simulink model "EPS_orbit_v1_R2019a"  (R2019a)
settings: Solver=FixedStepAuto  StartTime=0.0  StopTime=tsimulation  FixedStep=delta_t  RelTol=1e-3
values from neighbouring files (symbols this model uses):
  a = 6678    [demoEPS_R2019a.m]    (also in demoEPS_v1.m; demoEPS_v1a.m; demoEPS_v1test.m; demoEPS_v2.m)
  day = 21    [demoEPS_R2019a.m]    (also in demoEPS_v1.m = 1; demoEPS_v1a.m; demoEPS_v1test.m; demoEPS_v2.m)
  e = 0.001    [demoEPS_R2019a.m]    (also in demoEPS_v1.m = 0; demoEPS_v1a.m; demoEPS_v1test.m; demoEPS_v2.m)
  hours = 0    [demoEPS_R2019a.m]    (also in demoEPS_v1.m; demoEPS_v1a.m; demoEPS_v1test.m; demoEPS_v2.m)
  i = 51.6    [demoEPS_R2019a.m]    (also in demoEPS_v1.m; demoEPS_v1a.m; demoEPS_v1test.m; demoEPS_v2.m)
  m = 10    [demoEPS_R2019a.m]    (also in demoEPS_v1.m; demoEPS_v1a.m; demoEPS_v1test.m; demoEPS_v2.m)
  minutes = 0    [demoEPS_R2019a.m]    (also in demoEPS_v1.m; demoEPS_v1a.m; demoEPS_v1test.m; demoEPS_v2.m)
  month = 3    [demoEPS_R2019a.m]    (also in demoEPS_v1.m = 1; demoEPS_v1a.m = 6; demoEPS_v1test.m = 12; demoEPS_v2.m)
  nu = 0    [demoEPS_R2019a.m]    (also in demoEPS_v1.m; demoEPS_v1a.m; demoEPS_v1test.m; demoEPS_v2.m)
  O = 300    [demoEPS_R2019a.m]    (also in demoEPS_v1.m = 185; demoEPS_v1a.m = 69; demoEPS_v1test.m = 180; demoEPS_v2.m = 243)
  o = 90    [demoEPS_R2019a.m]    (also in demoEPS_v1.m; demoEPS_v1a.m = 150; demoEPS_v1test.m = 150; demoEPS_v2.m)
  Psa = 48    [demoEPS.m]    (also in demoEPS_R2019a.m; demoEPS_v1.m; demoEPS_v1a.m; demoEPS_v1test.m)
  seconds = 0    [demoEPS_R2019a.m]    (also in demoEPS_v1.m; demoEPS_v1a.m; demoEPS_v1test.m; demoEPS_v2.m)
  year = 2020    [demoEPS_R2019a.m]    (also in demoEPS_v1.m; demoEPS_v1a.m = 2019; demoEPS_v1test.m = 2019; demoEPS_v2.m)
undefined symbols (not defined in the file or in its folder): km, s
libraries: aerolibconvert2 x6, vrlib x5, dspmathops x2, aerolibutil x2, sharedtransform x1, aerolibgravity2 x1, aerolibcelestial x1
settings Model: Creator=Ricardo  LastModifiedBy=colpari

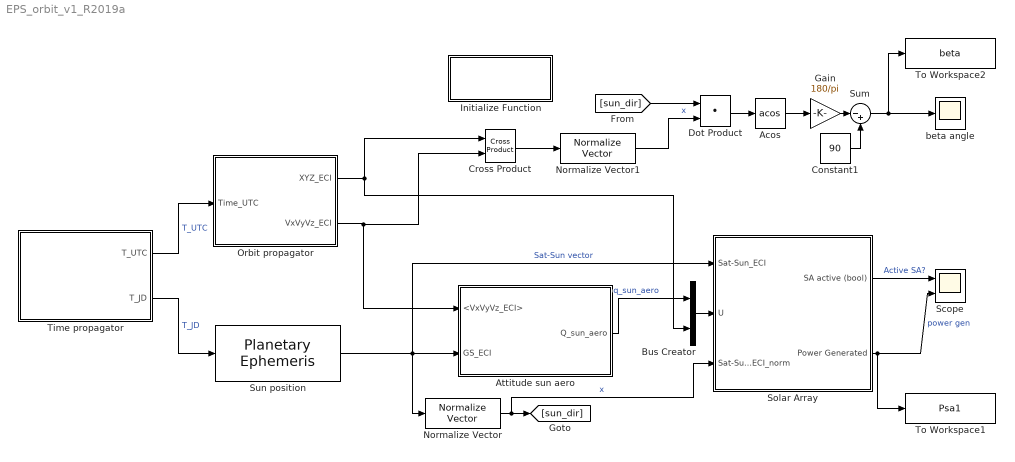
== system EPS_orbit_v1_R2019a ==
  Acos : Trigonometry  Operator=acos
  Attitude sun aero : Subsystem
  Bus Creator : BusCreator  Inputs=2
  Constant1 : Constant  Value=90
  Cross Product : vrlib/Utilities/Cross Product
  Dot Product : DotProduct  InputSameDT=on  OutDataTypeStr=Inherit: Inherit via internal rule
  Gain : Gain  Gain=180/pi
  Initialize Function : Subsystem  TreatAsAtomicUnit=on
  Normalize Vector : vrlib/Utilities/Normalize Vector  maxzero=0
  Normalize Vector1 : vrlib/Utilities/Normalize Vector  maxzero=0
  Orbit propagator : Subsystem
  Scope : Scope  NumInputPorts=2
  Solar Array : Subsystem
  Sum : Sum  Inputs=|-+
  Sun position : aerolibcelestial/Planetary Ephemeris  kmflag=km,km/s  epochflag=Julian date  de=DE405  nCenter=Earth  nTarget=Sun  errorflag=Error  velflag=off
      settings: SourceProductBaseCode=AE
  Time propagator : Subsystem
  To Workspace1 : ToWorkspace  VariableName=Psa1  SaveFormat=Timeseries  SampleTime=-1
  To Workspace2 : ToWorkspace  VariableName=beta  SaveFormat=Timeseries  SampleTime=-1
  beta angle : Scope
  wires:
  Orbit propagator/2(VxVyVz_ECI) -> Cross Product/2, Attitude sun aero/1(<VxVyVz_ECI>)
  Orbit propagator/1(XYZ_ECI) -> Cross Product/1, Bus Creator/2
  Normalize Vector/1 -> [sun_dir], Solar Array/3(Sat-Sun_ECI_norm)  "x"
  Bus Creator/1 -> Solar Array/2(U)
  Sun position/1 -> Normalize Vector/1, Solar Array/1(Sat-Sun_ECI), Attitude sun aero/2(GS_ECI)  "Sat-Sun vector"
  Solar Array/1(SA active (bool)) -> Scope/1  "Active SA?"
  Time propagator/1(T_UTC) -> Orbit propagator/1("Time_UTC ")  "T_UTC"
  Attitude sun aero/1(Q_sun_aero) -> Bus Creator/1  "q_sun_aero"
  Normalize Vector1/1 -> Dot Product/2  "x"
  Gain/1 -> Sum/1
  Solar Array/2(Power Generated) -> To Workspace1/1, Scope/2  "power gen"
  [sun_dir] -> Dot Product/1
  Acos/1 -> Gain/1
  Dot Product/1 -> Acos/1
  Time propagator/2(T_JD) -> Sun position/1  "T_JD"
  Cross Product/1 -> Normalize Vector1/1
  Sum/1 -> beta angle/1, To Workspace2/1
  Constant1/1 -> Sum/2

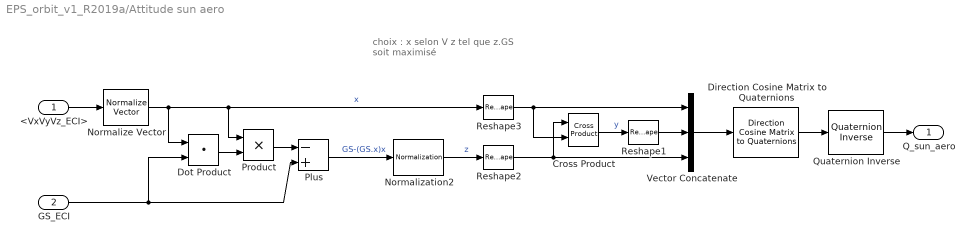
== system EPS_orbit_v1_R2019a/Attitude sun aero ==
  note: choix :
      | x selon V
      | z tel que z.GS soit maximisé
  <VxVyVz_ECI> : Inport
  GS_ECI : Inport  Port=2
  Cross Product : vrlib/Utilities/Cross Product
  Direction Cosine Matrix to Quaternions : sharedtransform/Direction Cosine Matrix  to Quaternions  aMode=0  action=None  tolerance=eps(2)
      settings: SourceProductBaseCode=AE,PW,MT,UV,VE,VP
  Dot Product : DotProduct  InputSameDT=on  OutDataTypeStr=Inherit: Inherit via internal rule
  Normalization2 : dspmathops/Normalization  NormType=2-norm  Bias=1e-10  NormOver=Each column  Dimension=1  roundingMode=Floor  overflowMode=off  accumDataTypeStr=Inherit: Same as product output  accumLastDataTypeStr=Inherit: Same as product output  outputDataTypeStr=Inherit: Same as product output  outputMin=[]  outputMax=[]  outputLastDataTypeStr=Inherit: Same as product output
  Normalize Vector : vrlib/Utilities/Normalize Vector  maxzero=0
  Plus : Sum  Inputs=-+
  Product : Product
  Quaternion Inverse : aerolibutil/Quaternion Inverse
  Reshape1 : Reshape  OutputDimensionality=Column vector (2-D)
  Reshape2 : Reshape  OutputDimensionality=Column vector (2-D)
  Reshape3 : Reshape  OutputDimensionality=Column vector (2-D)
  Vector Concatenate : Concatenate  NumInputs=3  Mode=Multidimensional array  ConcatenateDimension=2
  Q_sun_aero : Outport  VectorParamsAs1DForOutWhenUnconnected=off
  wires:
  Quaternion Inverse/1 -> Q_sun_aero/1
  Reshape2/1 -> Vector Concatenate/3, Cross Product/1
  Reshape3/1 -> Vector Concatenate/1, Cross Product/2
  Product/1 -> Plus/1
  Dot Product/1 -> Product/2
  Cross Product/1 -> Reshape1/1  "y"
  Normalization2/1 -> Reshape2/1  "z"
  Plus/1 -> Normalization2/1  "GS-(GS.x)x"
  GS_ECI/1 -> Dot Product/2, Plus/2
  Vector Concatenate/1 -> Direction Cosine Matrix to Quaternions/1
  Direction Cosine Matrix to Quaternions/1 -> Quaternion Inverse/1
  Normalize Vector/1 -> Dot Product/1, Product/1, Reshape3/1  "x"
  <VxVyVz_ECI>/1 -> Normalize Vector/1
  Reshape1/1 -> Vector Concatenate/2

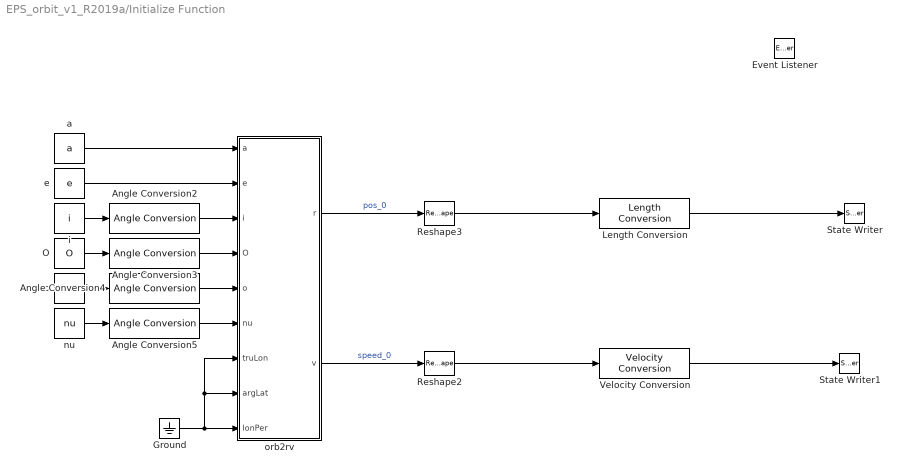
== system EPS_orbit_v1_R2019a/Initialize Function ==
  Angle Conversion{2..5} (4 alike) : aerolibconvert2/Angle Conversion  IU=deg  OU=rad
  Event Listener : EventListener  DisableCoverage=on  EventName=reset
  Ground : Ground
  Length Conversion : aerolibconvert2/Length Conversion  IU=km  OU=m
  O : Constant  Value=O
  Reshape2 : Reshape  OutputDimensionality=Column vector (2-D)
  Reshape3 : Reshape  OutputDimensionality=Column vector (2-D)
  State Writer : StateWriter  StateOwnerBlock=../../Orbit propagator/Integrator_pos
  State Writer1 : StateWriter  StateOwnerBlock=../../Orbit propagator/Integrator_speed
  Velocity Conversion : aerolibconvert2/Velocity Conversion  IU=km/s  OU=m/s
  a : Constant  Value=a
  e : Constant  Value=e
  i : Constant  Value=i
  nu : Constant  Value=nu
  o : Constant  Value=o
  orb2rv : MATLAB Function  TreatAsAtomicUnit=on
  wires:
  Angle Conversion2/1 -> orb2rv/3(i)
  Length Conversion/1 -> State Writer/1
  Angle Conversion4/1 -> orb2rv/5(o)
  nu/1 -> Angle Conversion5/1
  Angle Conversion3/1 -> orb2rv/4(O)
  e/1 -> orb2rv/2(e)
  Reshape3/1 -> Length Conversion/1
  O/1 -> Angle Conversion3/1
  a/1 -> orb2rv/1(a)
  i/1 -> Angle Conversion2/1
  orb2rv/1(r) -> Reshape3/1  "pos_0"
  o/1 -> Angle Conversion4/1
  Angle Conversion5/1 -> orb2rv/6(nu)
  Velocity Conversion/1 -> State Writer1/1
  Reshape2/1 -> Velocity Conversion/1
  orb2rv/2(v) -> Reshape2/1  "speed_0"
  Ground/1 -> orb2rv/8(argLat), orb2rv/7(truLon), orb2rv/9(lonPer)

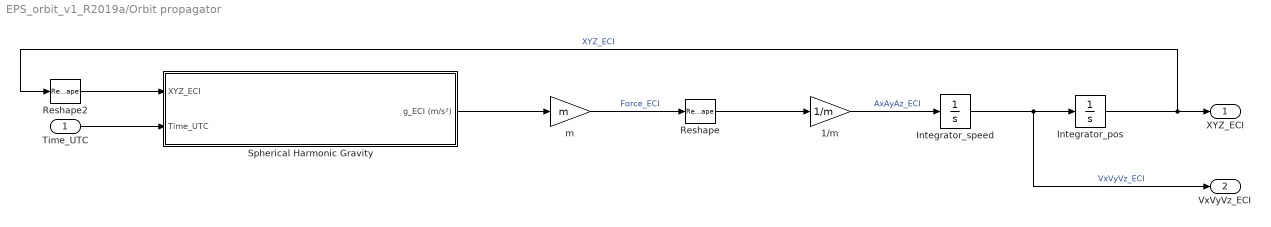
== system EPS_orbit_v1_R2019a/Orbit propagator ==
  "Time_UTC " : Inport
  1/m : Gain  Gain=1/m
  Integrator_pos : Integrator
  Integrator_speed : Integrator
  Reshape : Reshape  OutputDimensionality=Column vector (2-D)
  Reshape2 : Reshape  OutputDimensionality=Column vector (2-D)
  Spherical Harmonic Gravity : Subsystem  TreatAsAtomicUnit=on  SystemSampleTime=1
  m : Gain  Gain=m
  XYZ_ECI : Outport  VectorParamsAs1DForOutWhenUnconnected=off
  VxVyVz_ECI : Outport  Port=2
  wires:
  Integrator_pos/1 -> Reshape2/1, XYZ_ECI/1  "XYZ_ECI"
  Integrator_speed/1 -> VxVyVz_ECI/1, Integrator_pos/1  "VxVyVz_ECI"
  1/m/1 -> Integrator_speed/1  "AxAyAz_ECI"
  Reshape/1 -> 1/m/1
  m/1 -> Reshape/1  "Force_ECI"
  Spherical Harmonic Gravity/1(g_ECI (m/s²)) -> m/1
  "Time_UTC "/1 -> Spherical Harmonic Gravity/2(Time_UTC)
  Reshape2/1 -> Spherical Harmonic Gravity/1(XYZ_ECI)

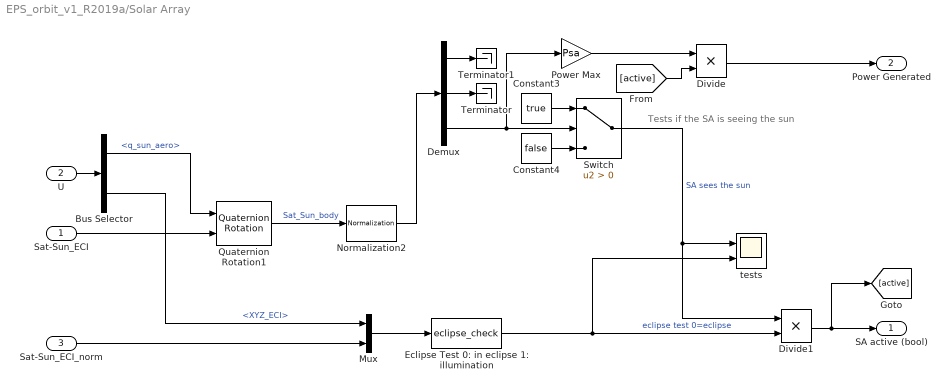
== system EPS_orbit_v1_R2019a/Solar Array ==
  note: Tests if the SA is seeing the sun
  Sat-Sun_ECI : Inport
  U : Inport  Port=2
  Sat-Sun_ECI_norm : Inport  Port=3
  Bus Selector : BusSelector  OutputSignals=q_sun_aero,XYZ_ECI
  Constant3 : Constant  Value=true
  Constant4 : Constant  Value=false
  Demux : Demux  Outputs=3
  Divide : Product  Inputs=**
  Divide1 : Product  Inputs=**
  Eclipse Test 0: in eclipse 1: illumination : MATLABFcn  MATLABFcn=eclipse_check
  Mux : Mux  Inputs=2
  Normalization2 : dspmathops/Normalization  NormType=2-norm  Bias=1e-10  NormOver=Each column  Dimension=1  roundingMode=Floor  overflowMode=off  accumDataTypeStr=Inherit: Same as product output  accumLastDataTypeStr=Inherit: Same as product output  outputDataTypeStr=Inherit: Same as product output  outputMin=[]  outputMax=[]  outputLastDataTypeStr=Inherit: Same as product output
  Power Max : Gain  Gain=Psa
  Quaternion Rotation1 : aerolibutil/Quaternion Rotation
  Switch : Switch  Criteria=u2 > Threshold
  Terminator : Terminator
  Terminator1 : Terminator
  tests : Scope  NumInputPorts=2
  SA active (bool) : Outport  VectorParamsAs1DForOutWhenUnconnected=off
  Power Generated : Outport  Port=2
  wires:
  Switch/1 -> Divide1/1, tests/1  "SA sees the sun"
  U/1 -> Bus Selector/1
  Sat-Sun_ECI/1 -> Quaternion Rotation1/2
  Bus Selector/1 -> Quaternion Rotation1/1  "<q_sun_aero>"
  Quaternion Rotation1/1 -> Normalization2/1  "Sat_Sun_body"
  Demux/3 -> Power Max/1, Switch/2
  Constant3/1 -> Switch/1
  Demux/2 -> Terminator/1
  Demux/1 -> Terminator1/1
  Bus Selector/2 -> Mux/1  "<XYZ_ECI>"
  Divide1/1 -> [active], SA active (bool)/1
  Constant4/1 -> Switch/3
  Normalization2/1 -> Demux/1
  Divide/1 -> Power Generated/1
  Power Max/1 -> Divide/1
  [active] -> Divide/2
  Sat-Sun_ECI_norm/1 -> Mux/2
  Mux/1 -> Eclipse Test 0: in eclipse 1: illumination/1
  Eclipse Test 0: in eclipse 1: illumination/1 -> tests/2, Divide1/2  "eclipse test 0=eclipse"

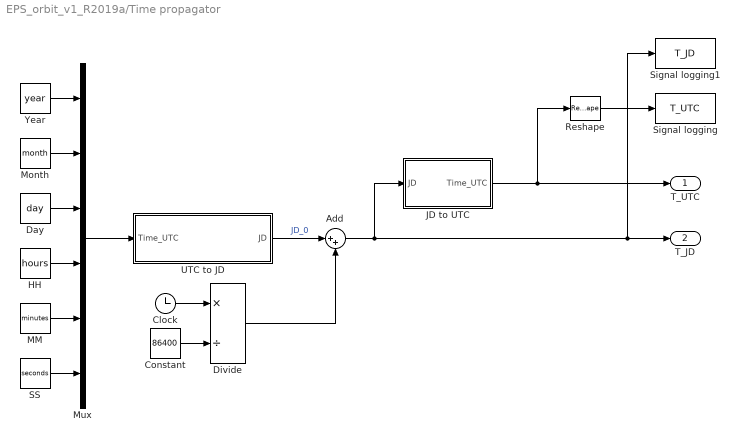
== system EPS_orbit_v1_R2019a/Time propagator ==
  Add : Sum  Inputs=|++
  Clock : Clock
  Constant : Constant  Value=86400
  Day : Constant  Value=day
  Divide : Product  Inputs=*/
  HH : Constant  Value=hours
  JD to UTC : MATLAB Function  TreatAsAtomicUnit=on
  MM : Constant  Value=minutes
  Month : Constant  Value=month
  Mux : Mux  Inputs=6
  Reshape : Reshape
  SS : Constant  Value=seconds
  Signal logging : ToWorkspace  VariableName=T_UTC  SaveFormat=Timeseries  SampleTime=1
      settings: Save2DSignal=2-D array (concatenate along first dimension)
  Signal logging1 : ToWorkspace  VariableName=T_JD  SaveFormat=Timeseries  SampleTime=1
      settings: Save2DSignal=2-D array (concatenate along first dimension)
  UTC to JD : MATLAB Function  TreatAsAtomicUnit=on
  Year : Constant  Value=year
  T_UTC : Outport  VectorParamsAs1DForOutWhenUnconnected=off
  T_JD : Outport  Port=2  VectorParamsAs1DForOutWhenUnconnected=off
  wires:
  UTC to JD/1(JD) -> Add/1  "JD_0"
  Clock/1 -> Divide/1
  Constant/1 -> Divide/2
  JD to UTC/1(Time_UTC) -> T_UTC/1, Reshape/1
  Divide/1 -> Add/2
  Mux/1 -> UTC to JD/1(Time_UTC)
  Day/1 -> Mux/3
  Month/1 -> Mux/2
  Year/1 -> Mux/1
  HH/1 -> Mux/4
  MM/1 -> Mux/5
  SS/1 -> Mux/6
  Reshape/1 -> Signal logging/1
  Add/1 -> Signal logging1/1, T_JD/1, JD to UTC/1(JD)

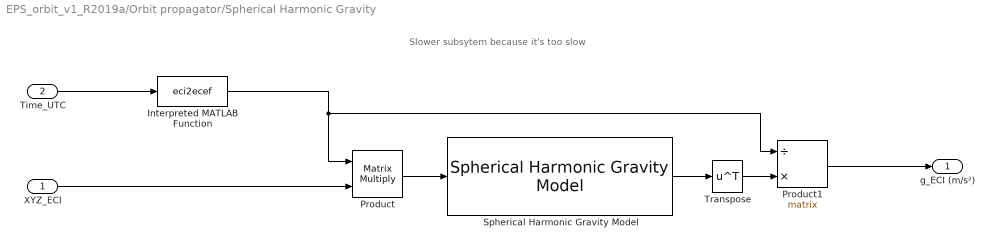
== system EPS_orbit_v1_R2019a/Orbit propagator/Spherical Harmonic Gravity ==
  note: Slower subsytem because it's too slow
  XYZ_ECI : Inport
  Time_UTC : Inport  Port=2
  Interpreted MATLAB Function : MATLABFcn  MATLABFcn=eci2ecef  OutputDimensions=[3;3]  Output1D=off
  Product : Product  Multiplication=Matrix(*)
  Product1 : Product  Inputs=/*  Multiplication=Matrix(*)
  Spherical Harmonic Gravity Model : aerolibgravity2/Spherical Harmonic Gravity Model  units=Metric (MKS)  degree=100  action=Warning  ptype=EGM2008  datafile='aerogmm2b.mat'
      settings: SourceProductBaseCode=AE
  Transpose : Math  Operator=transpose  SaturateOnIntegerOverflow=on
  g_ECI (m/s²) : Outport
  wires:
  Interpreted MATLAB Function/1 -> Product1/1, Product/1
  Transpose/1 -> Product1/2
  Product/1 -> Spherical Harmonic Gravity Model/1
  Spherical Harmonic Gravity Model/1 -> Transpose/1
  XYZ_ECI/1 -> Product/2
  Product1/1 -> g_ECI (m/s²)/1
  Time_UTC/1 -> Interpreted MATLAB Function/1

== matlab function EPS_orbit_v1_R2019a/Time propagator/JD to UTC ==
  data: JD input; Time_UTC output
function Time_UTC = fcn(JD)
    coder.extrinsic('datetime','datevec');
    Time_UTC = [0,0,0,0,0,0];
Time_UTC =  datevec(datetime(JD,'convertfrom','juliandate'));

== matlab function EPS_orbit_v1_R2019a/Time propagator/UTC to JD ==
  data: Time_UTC input; JD output
function JD = fcn(Time_UTC)

% JD = juliandate(Time_UTC);
JD = Dt2jD(Time_UTC);

== matlab function EPS_orbit_v1_R2019a/Initialize Function/orb2rv ==
  data: a input; r output; e input; i input; O input; o input; nu input; v output; truLon input; argLat input; lonPer input
%----------------------- Begin Code Sequence -----------------------------%
% Purpose:                                                                %
% Convert a given set of Keplerian Orbital Elements to state vectors in   %
% in the ECI frame of reference                                           %
%                                                                         %
%-------------------------------------------------------------------------%
%                                                                         %
% Inputs:                                                                 %
%-------- 
%a                      [1 x N]                         Semimajor axis
%                                                       (km)
%
%e                      [1 x N]                         Eccentricity Magnitude
%                                                       (unitless)
%
%i                      [1 x N]                         inclination
%                                                       (radians)
%
%O                      [1 x N]                         Right Ascention of
%                                                       the ascending node
%                                                       (radians)
%
%o                      [1 x N]                         Argument of perigee
%                                                       (radians)
%
%nu                     [1 x N]                         True Anomaly
%                                                       (radians)
%
%truLon                 [1 x N]                         True Longitude
%                                                       (radians)
%
%argLat                 [1 x N]                         Argument of Latitude
%                                                       (radians)
%
%lonPer                 [1 x N]                         Longitude of Periapse
%                                                       (radians)
%
%mu                     double                          Gravitational Constant
%                                                       Defaults to Earth if
%                                                       not specified
%
% Outputs:
%---------                                                                %
%r_ECI                  [3 x N]                         Position Vector in
%                                                       ECI coordinate
%                                                       frame of reference
%
%v_ECI                  [3 x N]                         Velocity vector in
%                                                       ECI coordinate
%                                                       frame of reference
%
% References:
%-------------
%Vallado,D. Fundamentals of Astrodynamics and Applications. 2007.
%
% Function Dependencies:
%------------------
%None
%------------------------------------------------------------------       %
% Programed by Darin Koblick  03-04-2012                                  %
%------------------------------------------------------------------       %
function [r,v] = orb2rv(a,e,i,O,o,nu,truLon,argLat,lonPer)
mu = 398600.4418;
%Make all inputs consistent w/ dimensions
a = a(:); e = e(:); i = i(:); O = O(:); o = o(:); nu = nu(:);
if e<1
    p=a*(1-e*e);
else
    p=2*a;
end
ietol = 1e-8;
idx = e < ietol & mod(i,pi) < ietol;
if any(idx); o(idx) = 0; O(idx) = 0; nu(idx) = truLon(idx); end
idx = e < ietol & mod(i,pi) > ietol;
if any(idx); o(idx) = 0; nu(idx) = argLat(idx); end
idx = e > ietol & mod(i,pi) < ietol;
if any(idx); O(idx) = 0; o(idx) = lonPer(idx); end
%Find rPQW and vPQW
rPQW = cat(2,p.*cos(nu)./(1 +e.*cos(nu)),p.*sin(nu)./(1+e.*cos(nu)),zeros(size(nu)));
vPQW = cat(2,-sqrt(mu./p).*sin(nu),sqrt(mu./p).*(e+cos(nu)),zeros(size(nu)));
%Create Transformation Matrix
PQW2IJK = NaN(3,3,size(p,1));
cO = cos(O); sO = sin(O); co = cos(o); so = sin(o); ci = cos(i); si = sin(i);
PQW2IJK(1,1,:) = cO.*co-sO.*so.*ci; PQW2IJK(1,2,:) = -cO.*so-sO.*co.*ci; PQW2IJK(1,3,:) = sO.*si;
PQW2IJK(2,1,:) = sO.*co+cO.*so.*ci; PQW2IJK(2,2,:) = -sO.*so+cO.*co.*ci; PQW2IJK(2,3,:) = -cO.*si;
PQW2IJK(3,1,:) = so.*si;            PQW2IJK(3,2,:) = co.*si;             PQW2IJK(3,3,:) = ci;
%Transform rPQW and vPQW to rECI and vECI
r = multiDimMatrixMultiply(PQW2IJK,rPQW)';  
v = multiDimMatrixMultiply(PQW2IJK,vPQW)';
end
function c = multiDimMatrixMultiply(a,b)
c = NaN(size(b));
c(:,1) = sum(bsxfun(@times,a(1,:,:),permute(b,[3 2 1])),2);
c(:,2) = sum(bsxfun(@times,a(2,:,:),permute(b,[3 2 1])),2);
c(:,3) = sum(bsxfun(@times,a(3,:,:),permute(b,[3 2 1])),2);
end
